simulink model "CIMA_SM"  (R2023b)
settings: Solver=VariableStepAuto  StartTime=0.0  StopTime=30  RelTol=1e-6
values from neighbouring files (symbols this model uses):
  a = 10    [CIMA_Classification_Stab_Equilibrium.m]    (also in CIMA_Control_routine.m)
  b = b_vec(i)    [CIMA_Classification_Stab_Equilibrium.m]    (also in CIMA_Control_routine.m = 2)
  x0 = [x1_eq+0.5; x2_eq+0.2]    [CIMA_Control_routine.m]
settings Model: Creator=user  LastModifiedBy=user
settings SolverCC: ZeroCrossAlgorithm=Adaptive
settings DataIOCC: SaveFormat=StructureWithTime
settings DebuggingCC: IgnoredZcDiagnostic=none

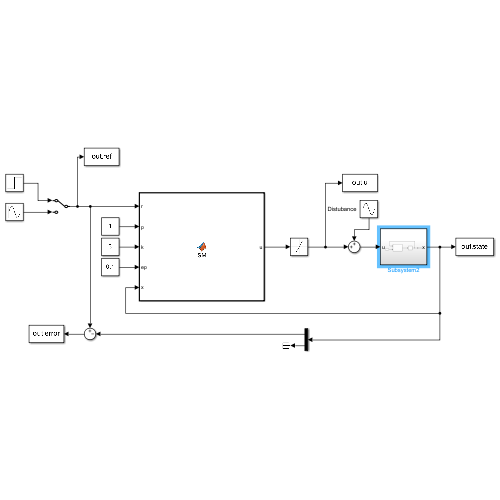
[thumbnail: Simulink's stored preview of the top-level diagram]
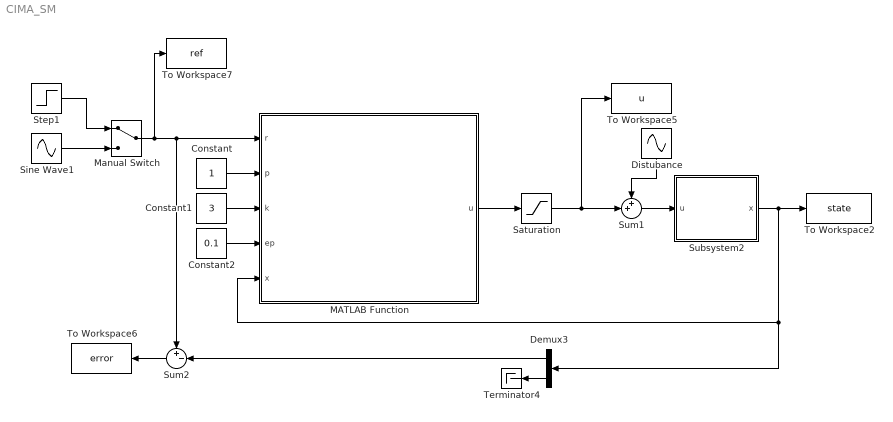
== system CIMA_SM ==
  Constant : Constant
  Constant1 : Constant  Value=3
  Constant2 : Constant  Value=0.1
  Demux3 : Demux  Outputs=2
  Distubance : Sin  Amplitude=0.3*0  SampleTime=0
  MATLAB Function : MATLAB Function  TreatAsAtomicUnit=on
  Manual Switch : ManualSwitch
  Saturation : Saturate  UpperLimit=20  LowerLimit=0
  Sine Wave1 : Sin  Amplitude=0.5  Bias=5  Frequency=2  SampleTime=0
  Step1 : Step  Time=0  After=5  SampleTime=0
  Subsystem2 : Subsystem
  Sum1 : Sum  Inputs=++|
  Sum2 : Sum  Inputs=+-|
  Terminator4 : Terminator
  To Workspace2 : ToWorkspace  VariableName=state  SaveFormat=Structure With Time  SampleTime=-1
  To Workspace5 : ToWorkspace  VariableName=u  SaveFormat=Structure With Time  SampleTime=-1
  To Workspace6 : ToWorkspace  VariableName=error  SaveFormat=Structure With Time  SampleTime=-1
  To Workspace7 : ToWorkspace  VariableName=ref  SaveFormat=Structure With Time  SampleTime=-1
  wires:
  Manual Switch/1 -> To Workspace7/1, Sum2/1, MATLAB Function/1(r)
  Subsystem2/1(x) -> Demux3/1, MATLAB Function/5(x), To Workspace2/1
  Demux3/2 -> Terminator4/1
  Step1/1 -> Manual Switch/1
  Sine Wave1/1 -> Manual Switch/2
  MATLAB Function/1(u) -> Saturation/1
  Saturation/1 -> To Workspace5/1, Sum1/2
  Constant/1 -> MATLAB Function/2(p)
  Constant1/1 -> MATLAB Function/3(k)
  Constant2/1 -> MATLAB Function/4(ep)
  Distubance/1 -> Sum1/1
  Sum1/1 -> Subsystem2/1(u)
  Demux3/1 -> Sum2/2
  Sum2/1 -> To Workspace6/1

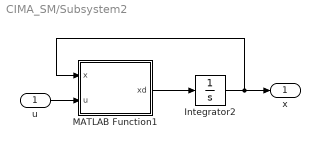
== system CIMA_SM/Subsystem2 ==
  u : Inport
  Integrator2 : Integrator  InitialCondition=x0  UpperSaturationLimit=18
  MATLAB Function1 : MATLAB Function  TreatAsAtomicUnit=on
  x : Outport
  wires:
  MATLAB Function1/1(xd) -> Integrator2/1
  Integrator2/1 -> x/1, MATLAB Function1/1(x)
  u/1 -> MATLAB Function1/2(u)

== matlab function CIMA_SM/MATLAB Function ==
  data: r input; p input; k input; ep input; a parameter; b parameter; u output; x input
function u  = SM(r, p, k, ep, a, b, x)

sigma = p*(x(1) - r);

Lf = p*(a - x(1) - (4*x(1)*x(2))/(1 + x(1)^2));
Lg = p;

u_eq = -Lf/Lg;

if abs(sigma) >= ep
   u_sw = sign(sigma);
else
   u_sw = sigma/ep;
end

u = -k/Lg*u_sw + u_eq;

== matlab function CIMA_SM/Subsystem2/MATLAB Function1 ==
  data: x input; u input; xd output; a parameter; b parameter
function xd = cima(x, u, a, b)

xd1 = a -x(1) - 4*x(1)*x(2)/(1 + x(1)^2) + u; 
xd2 = b*x(1)*(1 - x(2)/(1 + x(1)^2)); 

%Parameter uncertanties 10% 
%xd1 = 0.9*a -x(1) - 4*x(1)*x(2)/(1 + x(1)^2) + u; 
%xd2 = 1.1*b*x(1)*(1 - x(2)/(1 + x(1)^2)); 

%Parameter uncertanties 20% 
%xd1 = 1.2*a -x(1) - 4*x(1)*x(2)/(1 + x(1)^2) + u; 
%xd2 = 0.8*b*x(1)*(1 - x(2)/(1 + x(1)^2)); 

xd = [xd1;xd2];
